simulink model "UnitTestDebug"  (R2018b)
settings: Solver=FixedStepAuto  StartTime=0.0  StopTime=500  FixedStep=fswParams.sample_time_s  RelTol=1e-3
undefined symbols (not defined in the file or in its folder): DiscIntNeverNeededParam, fswParams, MEKF_lib, simParams, triad_coarse_estimator, TRIAD_coarse_estimator
libraries: vrlib x8, dspmathops x8, aerolibutil x7, simulink x6, sharedutil x3, sharedtransform x2, satelliteDynamics_lib x1
(part 2 of 2)

== matlab function UnitTestDebug/MEKF_lib/Time Propagation (q,P)/MATLAB Function10 ==
  data: om_mag input; omega_x input; dt input; Phi output
function Phi = Phi_disc(om_mag,omega_x,dt)
%#codegen
% State Transition Matrix
w_n     = om_mag;
w_skew  = omega_x;

if( w_n < 1e-10 )
    Phi = [ eye(3)     -eye(3)*dt;
            zeros(3,3)  eye(3) ];
else
    Phi_11  = eye(3) - w_skew*(sin(w_n*dt)/w_n) + ...
                                        w_skew^2*(1 - cos(w_n*dt))/w_n^2;
    Phi_12  = w_skew*(1 - cos(w_n*dt))/w_n^2 - eye(3)*dt - ...
                                    w_skew^2*(w_n*dt - sin(w_n*dt))/w_n^3;
    Phi_21  = zeros(3,3);    
    Phi_22  = eye(3);    
    Phi     = [ Phi_11 Phi_12;
                Phi_21 Phi_22 ];
end

== matlab function UnitTestDebug/MEKF_lib/Time Propagation (q,P)/MATLAB Function ==
  data: P_sq input; Phi_discrete input; P_sq output; Q_sq input
function P_sq  = Cqr(P_sq,Phi_discrete,Q_sq)
%#codegen

A_QR2 = [P_sq'*Phi_discrete';Q_sq'];
         [~,R2] = qr(A_QR2);
          sq_P_kp1 = R2(1:6,1:6)';
          P_sq = sq_P_kp1;
end

== matlab function UnitTestDebug/MEKF_lib/Measurement Update/P, Kalman Gain ==
  data: R input; Pplus output size=[6,6]; Pminus input; gyro_valid input; H input; K output size=[6,6]
function [Pplus,K] = fcn113(R,Pminus,gyro_valid,H)
K = Pminus*H'/(H*Pminus*H' + R);

if( gyro_valid == 0 )
    K(4:6,:) = zeros(3,6); %this is done so that we do not update bias based
                            % on false gyro readings
end

        KHI = (K*H - eye(6));
        Pplus= KHI*Pminus*KHI' + K*R*K';
end
